simulink model "KTH_pedestrian_autoware_cs"  (R2019a)
settings: Solver=ode5  StartTime=0.0  StopTime=15  FixedStep=1/300  RelTol=1e-3
PreLoadFcn:
  | mbxruntime.callbacks.PreLoadFcn(bdroot);
PostLoadFcn:
  | mbxruntime.callbacks.PostLoadFcn(bdroot);
InitFcn:
  | mbxruntime.callbacks.InitFcn(bdroot);
StartFcn:
  | mbxruntime.callbacks.StartFcn(bdroot);
StopFcn:
  | mbxruntime.callbacks.StopFcn(bdroot);
model workspace: external: MAT-File .\KTH_pedestrian_autoware_cs_hws.mat (data not in the file)
undefined symbols (not defined in the file or in its folder): DiscIntNeverNeededParam, InitImageOutputDir, KTH_pedestrian_autoware_cs_068c4cd025b302ec, KTH_pedestrian_autoware_cs_0912ea5e42e9497a, KTH_pedestrian_autoware_cs_1d9a8021db345c7c, KTH_pedestrian_autoware_cs_28872ec29a2665b0, KTH_pedestrian_autoware_cs_313ee8695bcfca2c, KTH_pedestrian_autoware_cs_3a67605991698ea5, KTH_pedestrian_autoware_cs_4351374c92dbfe8b, KTH_pedestrian_autoware_cs_610f55c1327f52b3, KTH_pedestrian_autoware_cs_6a3044fc88cecb81, KTH_pedestrian_autoware_cs_7342e95dd6ba7675, KTH_pedestrian_autoware_cs_75e80bfdb8f4de24, KTH_pedestrian_autoware_cs_7a295923ae4f036e, KTH_pedestrian_autoware_cs_b28d508533e0b342, KTH_pedestrian_autoware_cs_b6388f21b4a7e6a9, KTH_pedestrian_autoware_cs_bc2ee4423e8663e6, KTH_pedestrian_autoware_cs_c815ad16977e2770, KTH_pedestrian_autoware_cs_d476b555617a9f0e, KTH_pedestrian_autoware_cs_f89159477b4422a0, mbxruntime, tabledata
libraries: adeye_lib x16, PreScanSimulinkLibrary x6, PreScanUsefulBlocks x1, simulink x1
(part 1 of 4)
CloseFcn:
  | mbxruntime.callbacks.CloseFcn(bdroot);
settings Model: Creator=PRESCAN  LastModifiedBy=adeye
settings DataIOCC: LimitDataPoints=on  SaveFormat=Array  SignalLoggingSaveFormat=ModelDataLogs  ReturnWorkspaceOutputs=off
settings OptimizationCC: DefaultParameterBehavior=Inlined  ExpressionDepthLimit=2147483647  InitFltsAndDblsToZero=on  LifeSpan=inf
settings DebuggingCC: SaveWithParameterizedLinksMsg=none  UnderspecifiedInitializationDetection=Classic  MergeDetectMultiDrivingBlocksExec=none  SignalResolutionControl=TryResolveAllWithWarning  MultiTaskDSMMsg=warning  MultiTaskCondExecSysMsg=none  FcnCallInpInsideContextMsg=warning  StateNameClashWarn=warning  SFUnexpectedBacktrackingDiag=warning  SFNoUnconditionalDefaultTransitionDiag=warning  SFExecutionAtInitializationDiag=none  ArithmeticOperatorsInVariantConditions=warning
settings HardwareCC: ProdBitPerPointer=32  ProdBitPerSizeT=32  ProdBitPerPtrDiffT=32  ProdLargestAtomicFloat=None  ProdIntDivRoundTo=Undefined  ProdEndianess=Unspecified  ProdWordSize=32  ProdHWDeviceType=32-bit Generic
settings ModelReferenceCC: UpdateModelReferenceTargets=IfOutOfDate  PropagateSignalLabelsOutOfModel=off
settings SFSimCC: SimUseLocalCustomCode=off  SimParseCustomCode=off
settings SFSimCC: SimCustomHeaderCode=|
  | #include "prescan.h"
  | #include "prescan_platform.h"
settings RTWCC: RTWUseLocalCustomCode=off
settings CodeAppCC: StateflowObjectComments=on
settings GRTTargetCC: TargetFcnLib=ansi_tfl_tmw.mat  TargetLangStandard=C89/C90 (ANSI)  GeneratePreprocessorConditionals=Disable all  CombineOutputUpdateFcns=off  GRTInterface=on
settings ConfigComp: CovMetricSettings=dw  CovHtmlReporting=on  CovSaveCumulativeToWorkspaceVar=on  CovSaveSingleToWorkspaceVar=on  CovExternalEMLEnable=off  CovSFcnEnable=off

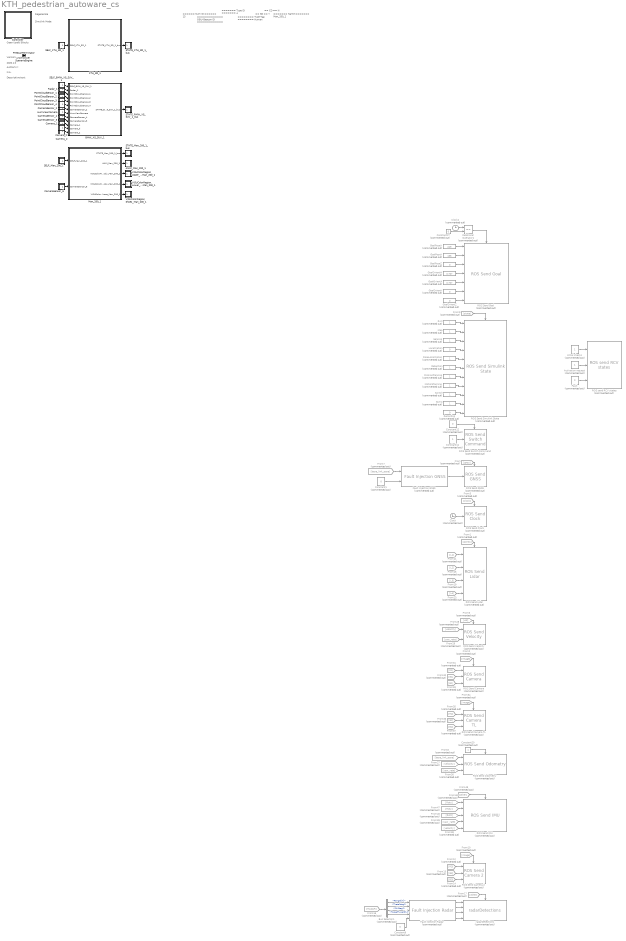
== system KTH_pedestrian_autoware_cs ==
  note: Regenerate
  note: Simulink Mode
  note: Open Useful Blocks
  note: 2020.1.0
  note: Version:
  note: Author(s):
  note: N.A.
  note: Descriptive text:
  note: ======
      | Num ID
      | ======
      | 13
  note: =============
      | OBU-Beacon ID
      | =============
  note: =======
      | Type ID
      | =======
      | 4
  note: ========
      | Type Tag
      | ========
      | Human
  note: ==
      | SD
      | ==
      | Y
  note: ==
      | CD
      | ==
      | N
  note: =======
      | Name
      | =======
      | Man_200_1
  ANIM_Man_200_1 : Subsystem  Tag=actuator/AnimationOutport  Priority=0  LoadFcn=load('PreScanAnimActuatorData.mat')  mask(PreScan Sink Block: State Animation){}
      mask help: The Human Animation port allows the human to walk, run or bend
      settings: OpenFcn=open_system([gcb '/Actuator'],'mask')
      mask Help: eval('openHelp(239)')
      mask Display: image(imread('HumanAnimated.jpg'))
  Activation request : Constant  Commented=on  OutDataTypeStr=Inherit: Inherit via back propagation
  BMW_X5_SUV_1 : Subsystem  Tag=WorldObjectSubSystem  InitFcn=UniqueId = '9040';
      mask init:
      | modelPath = GenericModelHelper.getGenericModelFilePath('ModelDepo','Vehicles\BMW_X5\BMW_X5.pgmb','bfeb1c11467705ab888b3011684c848b');imagePath = GenericModelHelper.getCompilationPicture(modelPath, 'BMW_X5_HighPoly.png');
      mask Display: image(imread(imagePath));color('white');text(0, 0, ' ID=23\n')
  Bus Selector1 : BusSelector  Commented=on  OutputSignals=Range[m],Theta[deg],Phi[deg],TargetTypeID[-]
  CameraSensor_2 : Subsystem  Tag=sensor/Camera/CameraSensor  Priority=30  mask(PreScan Source Block: Camera Sensor){}
      mask help: The Camera Sensor provides a color or monochrome image.
      settings: OpenFcn=open_system([gcb '/Sensor'],'mask')
      mask Help: eval('openHelp(457)')
      mask Display: image(imread('CameraSensor.png'))
  CameraSensor_3 : Subsystem  Tag=sensor/Camera/CameraSensor  Priority=30  mask(PreScan Source Block: Camera Sensor){}
      mask help: The Camera Sensor provides a color or monochrome image.
      settings: OpenFcn=open_system([gcb '/Sensor'],'mask')
      mask Help: eval('openHelp(457)')
      mask Display: image(imread('CameraSensor.png'))
  CameraSensor_4 : Subsystem  Tag=sensor/Camera/CameraSensor  Priority=30  mask(PreScan Source Block: Camera Sensor){}
      mask help: The Camera Sensor provides a color or monochrome image.
      settings: OpenFcn=open_system([gcb '/Sensor'],'mask')
      mask Help: eval('openHelp(457)')
      mask Display: image(imread('CameraSensor.png'))
  CameraSensor_6 : Subsystem  Tag=sensor/Camera/CameraSensor  Priority=30  mask(PreScan Source Block: Camera Sensor){}
      mask help: The Camera Sensor provides a color or monochrome image.
      settings: OpenFcn=open_system([gcb '/Sensor'],'mask')
      mask Help: eval('openHelp(457)')
      mask Display: image(imread('CameraSensor.png'))
  Camera_1 : Subsystem  Tag=sensor/Camera/CameraSensor  Priority=30  mask(PreScan Source Block: Camera Sensor){}
      mask help: The Camera Sensor provides a color or monochrome image.
      settings: OpenFcn=open_system([gcb '/Sensor'],'mask')
      mask Help: eval('openHelp(457)')
      mask Display: image(imread('CameraSensor.png'))
  Camera_2 : Subsystem  Tag=sensor/Camera/CameraSensor  Priority=30  mask(PreScan Source Block: Camera Sensor){}
      mask help: The Camera Sensor provides a color or monochrome image.
      settings: OpenFcn=open_system([gcb '/Sensor'],'mask')
      mask Help: eval('openHelp(457)')
      mask Display: image(imread('CameraSensor.png'))
  Camera_tl : Subsystem  Tag=sensor/Camera/CameraSensor  Priority=30  mask(PreScan Source Block: Camera Sensor){}
      mask help: The Camera Sensor provides a color or monochrome image.
      settings: OpenFcn=open_system([gcb '/Sensor'],'mask')
      mask Help: eval('openHelp(457)')
      mask Display: image(imread('CameraSensor.png'))
  Clock : Clock  Commented=on
  Clock2 : Clock  Commented=on
  Constant1 : Constant  Commented=on  Value=0  OutDataTypeStr=Inherit: Inherit via back propagation  SampleTime=0.05
  Constant11 : Constant  Commented=on  OutDataTypeStr=Inherit: Inherit via back propagation  SampleTime=0.05
  Constant12 : Constant  Commented=on  Value=0  OutDataTypeStr=Inherit: Inherit via back propagation  SampleTime=0.05
  Constant20 : Constant  Commented=on
  Constant27 : Constant  Commented=on  Value=0
  Constant9 : Constant  Commented=on  Value=0
  Controller : Subsystem  Description=8A3CD2955739A82C886C20AE3E253D78460D53180EE2C1B14CC08DF75A70BE77  Priority=-1  LoadFcn=load PreScanControllerData  mask(PreScan Simulation Controller){prescanversion='2020.1.0', ModelReferencing=off, TimeStep=1/300, ControlMode=0, PreScanExecutionMode=on, ControllerCount=0, ControllerIndex=0, ControllerOptions=''}
      mask prompts: prescanversion "PreScan Version"; ModelReferencing "Use Model Referencing"; TimeStep "Upload Period [s]"; ControlMode "Control Mode"; PreScanExecutionMode "Execution Mode"; ControllerCount "Controller Count"; ControllerIndex "Controller Index"; ControllerOptions "Controller Options"
      mask help:
      | Please do not remove this block from the compilation sheet,
      | as it connects the model to the PreScan environment.
      mask init:
      | model = bdroot(gcb);
      | ExperimentFile = mbxruntime.findExperimentFile(model,true); %relative path
      | 
      | [d1, d2, d3, prescandata] = prescan_Settings();
      | ModelDepo = fullfile(prescandata,'ModelDepo'); 
      | 
      | RTmode = mbxruntime.getRTMode(model);
      | 
      | SimulationMode = get_param(bdroot,'SimulationMode');
      | if strcmp(SimulationMode, 'rapid-accelerator')
      |     SimulationMode = 'external';
      | end
      | TargetName = get_param(bdroot,'SystemTargetFile');
      settings: ModelCloseFcn=assignin('base',['model_closed_' bdroot],true);
      mask Help: eval('openHelp(812)')
      mask Display: image(imread('prescanlogo.ico'))
  Detection : Constant  Commented=on
  FakeLocalization : Constant  Commented=on
  Fault : Constant  Commented=on  Value=0  OutDataTypeStr=Inherit: Inherit via back propagation
  Fault Injection GNSS : adeye_lib/Fault Injection GNSS  Commented=on  v=0.0001  f=20
  Fault Injection Radar : adeye_lib/Fault Injection Radar  Commented=on  n=7  vr=1  vt=1  vp=1
  From : From  Commented=on  GotoTag=gnss
  From1 : From  Commented=on  GotoTag=points
  From10 : From  Commented=on  GotoTag=image
  From11 : From  Commented=on  GotoTag=L1
  From12 : From  Commented=on  GotoTag=R3
  From13 : From  Commented=on  GotoTag=G3
  From14 : From  Commented=on  GotoTag=B3
  From15 : From  Commented=on  GotoTag=L2
  From16 : From  Commented=on  GotoTag=RADAR
  From17 : From  Commented=on  GotoTag=other  TagVisibility=global
  From19 : From  Commented=on  GotoTag=L3
  From2 : From  Commented=on  GotoTag=image
  From23 : From  Commented=on  GotoTag=L4
  From27 : From  Commented=on  GotoTag=velocity
  From28 : From  Commented=on  GotoTag=velocity
  From29 : From  Commented=on  GotoTag=yaw_rate
  From3 : From  Commented=on  GotoTag=clock
  From30 : From  Commented=on  GotoTag=yaw_rate
  From31 : From  Commented=on  GotoTag=R1
  From32 : From  Commented=on  GotoTag=G1
  From33 : From  Commented=on  GotoTag=B1
  From34 : From  Commented=on  GotoTag=image
  From35 : From  Commented=on  GotoTag=R2
  From36 : From  Commented=on  GotoTag=G2
  From37 : From  Commented=on  GotoTag=B2
  From38 : From  Commented=on  GotoTag=velocity
  From39 : From  Commented=on  GotoTag=yaw_rate
  From46 : From  Commented=on  GotoTag=Rotz
  From47 : From  Commented=on  GotoTag=Roty
  From48 : From  Commented=on  GotoTag=Rotx
  From49 : From  Commented=on  GotoTag=other  TagVisibility=global
  From5 : From  Commented=on  GotoTag=vel
  From7 : From  Commented=on  GotoTag=base_link_pose
  From8 : From  Commented=on  GotoTag=base_link_pose
  From9 : From  Commented=on  GotoTag=state
  GoalOrientW : Constant  Commented=on  Value=0.707
  GoalOrientX : Constant  Commented=on  Value=0.707
  GoalOrientY : Constant  Commented=on  Value=0
  GoalOrientZ : Constant  Commented=on  Value=0
  GoalPoseX : Constant  Commented=on  Value=249
  GoalPoseY : Constant  Commented=on  Value=136
  GoalPoseZ : Constant  Commented=on  Value=0
  HumViewCamera : Subsystem  Tag=sensor/Camera/CameraSensor  Priority=30  mask(PreScan Source Block: Camera Sensor){}
      mask help: The Camera Sensor provides a color or monochrome image.
      settings: OpenFcn=open_system([gcb '/Sensor'],'mask')
      mask Help: eval('openHelp(457)')
      mask Display: image(imread('CameraSensor.png'))
  Initial checks : Constant  Commented=on  OutDataTypeStr=Inherit: Inherit via back propagation
  KTH_3D_1 : Subsystem  Tag=WorldObjectSubSystem  InitFcn=UniqueId = '14987';
      mask init:
      | imagePath=which('KTH_3D.jpg');
      mask Display: image(imread(imagePath));color('white');text(0, 0, ' ID=14\n')
  Localization : Constant  Commented=on  Value=0
  Man_200_1 : Subsystem  Tag=WorldObjectSubSystem  InitFcn=UniqueId = '20104';
      mask init:
      | modelPath = GenericModelHelper.getGenericModelFilePath('ModelDepo','Humans\Male200\Male_200.pgmb','97a2394f555eb1924c7e25baff3f8b80');imagePath = GenericModelHelper.getCompilationPicture(modelPath, 'Male200.png');
      mask Display: image(imread(imagePath));color('white');text(0, 0, ' ID=13\n')
  Map : Constant  Commented=on
  MissionPlanning : Constant  Commented=on
  MotionPlanning : Constant  Commented=on
  PointCloudSensor_1 : Subsystem  Tag=sensor/PointCloudInport  Priority=30  mask(PreScan Source Block: Point Cloud Sensor){}
      mask help: The Point Cloud Sensor provides XYZ positions relative to the sensor
      settings: OpenFcn=open_system([gcb '/Sensor'],'mask')
      mask Help: eval('openHelp(6400)')
      mask Display: image(imread('PointCloudSensorSL.png'))
  PointCloudSensor_2 : Subsystem  Tag=sensor/PointCloudInport  Priority=30  mask(PreScan Source Block: Point Cloud Sensor){}
      mask help: The Point Cloud Sensor provides XYZ positions relative to the sensor
      settings: OpenFcn=open_system([gcb '/Sensor'],'mask')
      mask Help: eval('openHelp(6400)')
      mask Display: image(imread('PointCloudSensorSL.png'))
  PointCloudSensor_3 : Subsystem  Tag=sensor/PointCloudInport  Priority=30  mask(PreScan Source Block: Point Cloud Sensor){}
      mask help: The Point Cloud Sensor provides XYZ positions relative to the sensor
      settings: OpenFcn=open_system([gcb '/Sensor'],'mask')
      mask Help: eval('openHelp(6400)')
      mask Display: image(imread('PointCloudSensorSL.png'))
  PointCloudSensor_4 : Subsystem  Tag=sensor/PointCloudInport  Priority=30  mask(PreScan Source Block: Point Cloud Sensor){}
      mask help: The Point Cloud Sensor provides XYZ positions relative to the sensor
      settings: OpenFcn=open_system([gcb '/Sensor'],'mask')
      mask Help: eval('openHelp(6400)')
      mask Display: image(imread('PointCloudSensorSL.png'))
  PreScanTerminator : Subsystem  Tag=PreScanTerminator  Priority=999  LoadFcn=load PrescanTerminatorData  mask(PreScan Simulation Terminator){TimeStep=1/300}
      mask prompts: TimeStep "Upload Period [s]"
      mask help:
      | Please do not remove this block from the compilation sheet as it
      | connects the model to the PreScan environment.
      mask Help: eval('openHelp(812)')
      mask Display: image(imread('prescanlogo.ico'))
  ROS Send Camera : adeye_lib/ROS Send Camera  Commented=on  SystemSampleTime=-1
  ROS Send Camera 2 : adeye_lib/ROS Send Camera 2  Commented=on  SystemSampleTime=-1
  ROS Send Camera TL : adeye_lib/ROS Send Camera TL  Commented=on  SystemSampleTime=-1
  ROS Send Clock : adeye_lib/ROS Send Clock  Commented=on  SystemSampleTime=-1
  ROS Send GNSS : adeye_lib/ROS Send GNSS  Commented=on  SystemSampleTime=-1
  ROS Send Goal : adeye_lib/ROS Send Goal  Commented=on  SystemSampleTime=-1
  ROS Send IMU : adeye_lib/ROS Send IMU  Commented=on  SystemSampleTime=-1
  ROS Send Lidar : adeye_lib/ROS Send Lidar  Commented=on  SystemSampleTime=-1
  ROS Send Odometry : adeye_lib/ROS Send Odometry  Commented=on  SystemSampleTime=-1
  ROS Send Simulink State : adeye_lib/ROS Send Simulink State  Commented=on  SystemSampleTime=-1
  ROS Send Switch Command : adeye_lib/ROS Send Switch Command  Commented=on  SystemSampleTime=-1
  ROS Send Velocity : adeye_lib/ROS Send Velocity  Commented=on  SystemSampleTime=-1
  ROS send RCV states : adeye_lib/ROS send RCV states  Commented=on  SystemSampleTime=-1
  Radar_1 : Subsystem  Tag=sensor/Radar  Priority=30  LoadFcn=load('PrescanScannerSensorData.mat');load('PrescanScannerSensorMessage.mat')  mask(PreScan Source Block: Radar Sensor){}
      mask help:
      | The Radar Sensor is a detailed sensor based on a physical radar
      | model that includes Antenna GAIN Maps (AGM) and atmospheric
      | attenuation.
      |
      | For more information, please click Help.
      settings: OpenFcn=open_system([gcb '/Sensor'],'mask')
      mask Help: eval('openHelp(1464)')
      mask Display: image(imread('Radar.png'))
  Recording : Constant  Commented=on  Value=0
  Relational Operator1 : RelationalOperator  Commented=on  Operator===  OutDataTypeStr=boolean  RndMeth=Simplest
  Rviz : Constant  Commented=on
  SELF_BMW_X5_SUV_1 : Subsystem  Tag=sensor/SelfPort  Priority=30  LoadFcn=load('PreScanSelfSensorData.mat')  mask(PreScan Source Block: SELF){}
      mask help:
      | The SELF port shows (state) information of the actor itself. The outputs are position in the experiment's axis system and the GPS coordinates, and the object's absolute velocity and compass heading.
      |
      | For more information, please click Help.
      settings: OpenFcn=open_system([gcb '/Sensor'],'mask')
      mask Help: eval('openHelp(462)')
      mask Display: image(imread('GPS.png'))
  SELF_KTH_3D_1 : Subsystem  Tag=sensor/SelfPort  Priority=30  LoadFcn=load('PreScanSelfSensorData.mat')  mask(PreScan Source Block: SELF){}
      mask help:
      | The SELF port shows (state) information of the actor itself. The outputs are position in the experiment's axis system and the GPS coordinates, and the object's absolute velocity and compass heading.
      |
      | For more information, please click Help.
      settings: OpenFcn=open_system([gcb '/Sensor'],'mask')
      mask Help: eval('openHelp(462)')
      mask Display: image(imread('GPS.png'))
  SELF_Man_200_1 : Subsystem  Tag=sensor/SelfPort  Priority=30  LoadFcn=load('PreScanSelfSensorData.mat')  mask(PreScan Source Block: SELF){}
      mask help:
      | The SELF port shows (state) information of the actor itself. The outputs are position in the experiment's axis system and the GPS coordinates, and the object's absolute velocity and compass heading.
      |
      | For more information, please click Help.
      settings: OpenFcn=open_system([gcb '/Sensor'],'mask')
      mask Help: eval('openHelp(462)')
      mask Display: image(imread('GPS.png'))
  STATE_BMW_X5_SUV_1_bus : Subsystem  Tag=actuator/StatePort  Priority=0  LoadFcn=load('PreScanStateActuatorData.mat')  mask(PreScan Sink Block: State){}
      mask help:
      | The Actor State contains a vector signal of size (9x1), containing the following signals:
      |
      | -  Position    	(x,y,z)             	[m]
      | -  Velocity    	(vx,vy,vz)         	[m/s]
      | -  Angles       	(Roll, Pitch, Yaw)	[rad]
      |
      | The Actor state is defined in the global axis system.
      | The state is superponed on the Initial position defined in the GUI.
      |
      | For more information, please click Help.
      settings: OpenFcn=open_system([gcb '/Actuator'],'mask')
      mask Help: eval('openHelp(222)')
      mask Display: image(imread('State.png'))
  STATE_KTH_3D_1_bus : Subsystem  Tag=actuator/StatePort  Priority=0  LoadFcn=load('PreScanStateActuatorData.mat')  mask(PreScan Sink Block: State){}
      mask help:
      | The Actor State contains a vector signal of size (9x1), containing the following signals:
      |
      | -  Position    	(x,y,z)             	[m]
      | -  Velocity    	(vx,vy,vz)         	[m/s]
      | -  Angles       	(Roll, Pitch, Yaw)	[rad]
      |
      | The Actor state is defined in the global axis system.
      | The state is superponed on the Initial position defined in the GUI.
      |
      | For more information, please click Help.
      settings: OpenFcn=open_system([gcb '/Actuator'],'mask')
      mask Help: eval('openHelp(222)')
      mask Display: image(imread('State.png'))
  STATE_Man_200_1_bus : Subsystem  Tag=actuator/StatePort  Priority=0  LoadFcn=load('PreScanStateActuatorData.mat')  mask(PreScan Sink Block: State){}
      mask help:
      | The Actor State contains a vector signal of size (9x1), containing the following signals:
      |
      | -  Position    	(x,y,z)             	[m]
      | -  Velocity    	(vx,vy,vz)         	[m/s]
      | -  Angles       	(Roll, Pitch, Yaw)	[rad]
      |
      | The Actor state is defined in the global axis system.
      | The state is superponed on the Initial position defined in the GUI.
      |
      | For more information, please click Help.
      settings: OpenFcn=open_system([gcb '/Actuator'],'mask')
      mask Help: eval('openHelp(222)')
      mask Display: image(imread('State.png'))
  ScenarioEngine : Subsystem  Tag=PreScanOpenScenarioBlock  Priority=10  LoadFcn=load PrescanSynchronizeData  mask(PreScan Simulation Core Block){TimeStep=1/300}
      mask prompts: TimeStep "Timestep [s]"
      mask help:
      | Please do not remove this block from the PreScan compilation sheet,
      | as it contains essential configuration parameters for a PreScan simulation.
      settings: DeleteFcn=PreScanBlockDeleteFcn;
      mask Display: image(imread('prescanlogo.ico'))
  Sensing : Constant  Commented=on
  Ssmp : Constant  Commented=on
  Switch : Constant  Commented=on
  Synchronizer : Subsystem  Tag=PreScanSynchronizer  Priority=20  LoadFcn=load PrescanSynchronizeData  mask(PreScan Simulation Core Block){TimeStep=1/300}
      mask prompts: TimeStep "Timestep [s]"
      mask help:
      | Please do not remove this block from the PreScan compilation sheet,
      | as it contains essential configuration parameters for a PreScan simulation.
      settings: DeleteFcn=PreScanBlockDeleteFcn;
      mask Display: image(imread('prescanlogo.ico'))
  VISUColorRegion_Lower_Body_Man_200_1 : Subsystem  Tag=actuator/ColorRegion  Priority=0  LoadFcn=load('PrescanColorData')  mask(PreScan Sink Block: VisuTextureColor){}
      mask help:
      | The VisuTextureColor block provides a way to adapt the color of a vehicle.
      |
      | For more information, please click Help.
      settings: OpenFcn=open_system([gcb '/Actuator'],'mask')
      mask Help: eval('openHelp(230)')
      mask Display: image(imread('TextureColor.png'))
  VISUColorRegion_Shoes_Man_200_1 : Subsystem  Tag=actuator/ColorRegion  Priority=0  LoadFcn=load('PrescanColorData')  mask(PreScan Sink Block: VisuTextureColor){}
      mask help:
      | The VisuTextureColor block provides a way to adapt the color of a vehicle.
      |
      | For more information, please click Help.
      settings: OpenFcn=open_system([gcb '/Actuator'],'mask')
      mask Help: eval('openHelp(230)')
      mask Display: image(imread('TextureColor.png'))
  VISUColorRegion_Upper_Body_Man_200_1 : Subsystem  Tag=actuator/ColorRegion  Priority=0  LoadFcn=load('PrescanColorData')  mask(PreScan Sink Block: VisuTextureColor){}
      mask help:
      | The VisuTextureColor block provides a way to adapt the color of a vehicle.
      |
      | For more information, please click Help.
      settings: OpenFcn=open_system([gcb '/Actuator'],'mask')
      mask Help: eval('openHelp(230)')
      mask Display: image(imread('TextureColor.png'))
  radarDetections : adeye_lib/radarDetections  Commented=on  SystemSampleTime=-1
  wires:
  Activation request/1 -> ROS send RCV states/2
  Initial checks/1 -> ROS send RCV states/1
  Fault/1 -> ROS send RCV states/3
  GoalOrientY/1 -> ROS Send Goal/6
  Recording/1 -> ROS Send Simulink State/11
  Constant12/1 -> ROS Send Switch Command/Enable
  Relational Operator1/1 -> ROS Send Goal/Enable
  From33/1 -> ROS Send Camera/3
  GoalOrientW/1 -> ROS Send Goal/4
  Fault Injection Radar/1 -> radarDetections/1
  Constant1/1 -> Fault Injection GNSS/2
  Fault Injection Radar/2 -> radarDetections/2
  From3/1 -> ROS Send Clock/Enable
  GoalOrientX/1 -> ROS Send Goal/5
  From9/1 -> ROS Send Simulink State/Enable
  From37/1 -> ROS Send Camera TL/3
  From31/1 -> ROS Send Camera/1
  From49/1 -> ROS Send IMU/Enable
  From39/1 -> ROS Send IMU/4
  GoalPoseY/1 -> ROS Send Goal/2
  From48/1 -> ROS Send IMU/1
  From14/1 -> ROS Send Camera 2/3
  Bus Selector1/2 -> Fault Injection Radar/2  "<Theta[deg]>"
  From/1 -> ROS Send GNSS/Enable
  Fault Injection GNSS/1 -> ROS Send GNSS/1
  From36/1 -> ROS Send Camera TL/2
  From35/1 -> ROS Send Camera TL/1
  Sensing/1 -> ROS Send Simulink State/3
  GoalPoseZ/1 -> ROS Send Goal/3
  From19/1 -> ROS Send Lidar/3
  From16/1 -> Bus Selector1/1
  GoalPoseX/1 -> ROS Send Goal/1
  From15/1 -> ROS Send Lidar/2
  From11/1 -> ROS Send Lidar/1
  From28/1 -> ROS Send Velocity/1
  From46/1 -> ROS Send IMU/3
  Clock2/1 -> Relational Operator1/1
  Clock/1 -> ROS Send Clock/1
  From32/1 -> ROS Send Camera/2
  From38/1 -> ROS Send IMU/5
  From34/1 -> ROS Send Camera TL/Enable
  From13/1 -> ROS Send Camera 2/2
  From10/1 -> ROS Send Camera 2/Enable
  From29/1 -> ROS Send Velocity/2
  From8/1 -> ROS Send Odometry/1
  From5/1 -> ROS Send Velocity/Enable
  Fault Injection Radar/3 -> radarDetections/3
  From7/1 -> Fault Injection GNSS/1
  From23/1 -> ROS Send Lidar/4
  From1/1 -> ROS Send Lidar/Enable
  MotionPlanning/1 -> ROS Send Simulink State/8
  GoalOrientZ/1 -> ROS Send Goal/7
  FakeLocalization/1 -> ROS Send Simulink State/5
  MissionPlanning/1 -> ROS Send Simulink State/7
  Bus Selector1/4 -> Fault Injection Radar/4  "<TargetTypeID[-]>"
  Localization/1 -> ROS Send Simulink State/4
  Rviz/1 -> ROS Send Simulink State/1
  Map/1 -> ROS Send Simulink State/2
  From47/1 -> ROS Send IMU/2
  From2/1 -> ROS Send Camera/Enable
  Bus Selector1/1 -> Fault Injection Radar/1  "<Range[m]>"
  Detection/1 -> ROS Send Simulink State/6
  Constant27/1 -> Relational Operator1/2
  Ssmp/1 -> ROS Send Simulink State/10
  From12/1 -> ROS Send Camera 2/1
  From30/1 -> ROS Send Odometry/3
  From27/1 -> ROS Send Odometry/2
  Fault Injection Radar/4 -> radarDetections/4
  Switch/1 -> ROS Send Simulink State/9
  Constant9/1 -> Fault Injection Radar/5
  Constant11/1 -> ROS Send Switch Command/1
  Bus Selector1/3 -> Fault Injection Radar/3  "<Phi[deg]>"
  Constant20/1 -> ROS Send Odometry/Enable
  From17/1 -> radarDetections/Enable
  KTH_3D_1/1(STATE_KTH_3D_1_bus) -> STATE_KTH_3D_1_bus/1(STATE_KTH_3D_1_bus)
  SELF_KTH_3D_1/1(SELF_KTH_3D_1) -> KTH_3D_1/1(SELF_KTH_3D_1)
  BMW_X5_SUV_1/1(STATE_BMW_X5_SUV_1_bus) -> STATE_BMW_X5_SUV_1_bus/1(STATE_BMW_X5_SUV_1_bus)
  SELF_BMW_X5_SUV_1/1(SELF_BMW_X5_SUV_1) -> BMW_X5_SUV_1/1(SELF_BMW_X5_SUV_1)
  Radar_1/1(Radar_1) -> BMW_X5_SUV_1/2(Radar_1)
  PointCloudSensor_1/1(PointCloudSensor_1) -> BMW_X5_SUV_1/3(PointCloudSensor_1)
  PointCloudSensor_2/1(PointCloudSensor_2) -> BMW_X5_SUV_1/4(PointCloudSensor_2)
  PointCloudSensor_3/1(PointCloudSensor_3) -> BMW_X5_SUV_1/5(PointCloudSensor_3)
  PointCloudSensor_4/1(PointCloudSensor_4) -> BMW_X5_SUV_1/6(PointCloudSensor_4)
  CameraSensor_2/1(CameraSensor_2) -> BMW_X5_SUV_1/7(CameraSensor_2)
  HumViewCamera/1(HumViewCamera) -> BMW_X5_SUV_1/8(HumViewCamera)
  CameraSensor_4/1(CameraSensor_4) -> BMW_X5_SUV_1/9(CameraSensor_4)
  CameraSensor_3/1(CameraSensor_3) -> BMW_X5_SUV_1/10(CameraSensor_3)
  Camera_1/1(Camera_1) -> BMW_X5_SUV_1/11(Camera_1)
  Camera_tl/1(Camera_tl) -> BMW_X5_SUV_1/12(Camera_tl)
  Camera_2/1(Camera_2) -> BMW_X5_SUV_1/13(Camera_2)
  Man_200_1/1(STATE_Man_200_1_bus) -> STATE_Man_200_1_bus/1(STATE_Man_200_1_bus)
  Man_200_1/2(ANIM_Man_200_1) -> ANIM_Man_200_1/1(ANIM_Man_200_1)
  SELF_Man_200_1/1(SELF_Man_200_1) -> Man_200_1/1(SELF_Man_200_1)
  CameraSensor_6/1(CameraSensor_6) -> Man_200_1/2(CameraSensor_6)
  Man_200_1/3(VISUColorRegion_Upper_Body_Man_200_1) -> VISUColorRegion_Upper_Body_Man_200_1/1(VISUColorRegion_Upper_Body_Man_200_1)
  Man_200_1/4(VISUColorRegion_Lower_Body_Man_200_1) -> VISUColorRegion_Lower_Body_Man_200_1/1(VISUColorRegion_Lower_Body_Man_200_1)
  Man_200_1/5(VISUColorRegion_Shoes_Man_200_1) -> VISUColorRegion_Shoes_Man_200_1/1(VISUColorRegion_Shoes_Man_200_1)

== system KTH_pedestrian_autoware_cs/ANIM_Man_200_1 ==
  ANIM_Man_200_1 : Inport  Tag=inport/AnimationOutport  OutDataTypeStr=Bus: PRESCAN_ANIMACTUATORDATA  PortDimensions=1  SampleTime=1/300  BusOutputAsStruct=on
  Actuator : S-Function  FunctionName=sfun_AnimActuator  Parameters=UniqueID, TimeStep  SFunctionDeploymentMode=off  EnableBusSupport=off  mask(PreScan Sink Block: State Animation){UniqueID=20104, TimeStep=1/300}
      mask prompts: UniqueID "Auto-Assigned: Unique ID"; TimeStep "Auto-Assigned: Upload Period [s]"
      mask help: The Human Animation port allows the human to walk, run or bend
      mask Help: eval('openHelp(239)')
      mask Display: image(imread('HumanAnimated.jpg'))
  wires:
  ANIM_Man_200_1/1 -> Actuator/1
